simulink model "GMSK"  (R2024a)
settings: Solver=VariableStepAuto  StartTime=0.0  StopTime=4e-5  RelTol=1e-3
undefined symbols (not defined in the file or in its folder): DESIGN_CONST
libraries: dspfdesign x5, simulink x2, dspsigops x1, msbPllFoundation x1
settings Model: Creator=Sayantan  LastModifiedBy=Sayantan

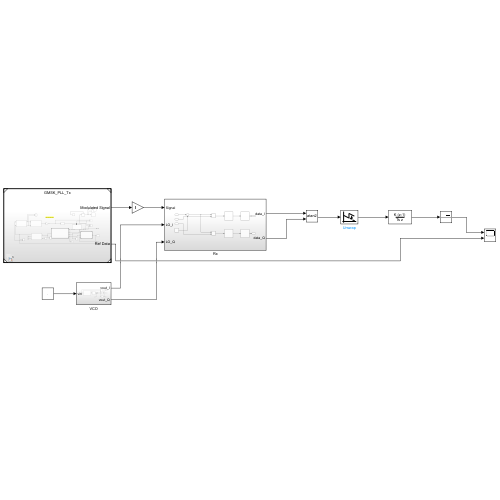
[thumbnail: Simulink's stored preview of the top-level diagram]
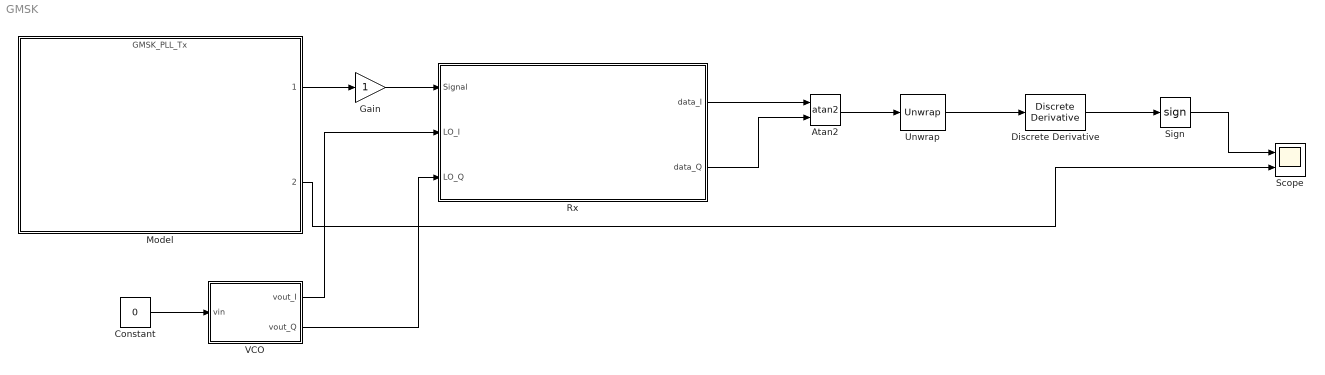
== system GMSK ==
  Atan2 : Trigonometry  Operator=atan2
  Constant : Constant  Value=0
  Discrete Derivative : simulink/Discrete/Discrete Derivative  gainval=1.0  ICPrevScaledInput=0.0  OutMin=[]  OutMax=[]  OutDataType=fixdt(1, 16)  OutScaling=2^-10  DoSatur=off
  Gain : Gain
  Model : ModelReference  ModelNameDialog=GMSK_PLL_Tx.slx  SimulationMode=Normal  ModelReferenceVersion=1.48
  Rx : Subsystem
  Scope : Scope  NumInputPorts=2
  Sign : Signum
  Unwrap : dspsigops/Unwrap  tol=pi  InputProcessing=Columns as channels (frame based)  running=off
  VCO : Subsystem
  wires:
  Gain/1 -> Rx/1(Signal)
  Model/1 -> Gain/1
  VCO/1(vout_I) -> Rx/2(LO_I)
  VCO/2(vout_Q) -> Rx/3(LO_Q)
  Model/2 -> Scope/2
  Rx/1(data_I) -> Atan2/1
  Rx/2(data_Q) -> Atan2/2
  Constant/1 -> VCO/1(vin)
  Atan2/1 -> Unwrap/1
  Sign/1 -> Scope/1
  Unwrap/1 -> Discrete Derivative/1
  Discrete Derivative/1 -> Sign/1

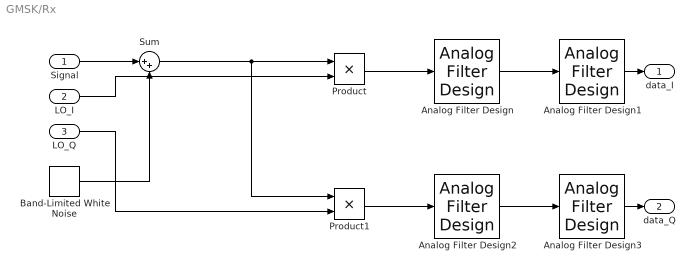
== system GMSK/Rx ==
  Signal : Inport
  LO_I : Inport  Port=2
  LO_Q : Inport  Port=3
  Analog Filter Design{,1..3} (4 alike) : dspfdesign/Analog Filter Design  method=Butterworth  filttype=Lowpass  N=1  Wlo=2*pi*(5e6)  Whi=80  Rp=2  Rs=40
  Band-Limited White Noise : simulink/Sources/Band-Limited White Noise  Cov=[0]  Ts=DESIGN_CONST.Tsim  seed=[23341]
  Product : Product
  Product1 : Product
  Sum : Sum  Inputs=|++
  data_I : Outport
  data_Q : Outport  Port=2
  wires:
  Analog Filter Design1/1 -> data_I/1
  Sum/1 -> Product1/1, Product/1
  Analog Filter Design/1 -> Analog Filter Design1/1
  Product/1 -> Analog Filter Design/1
  Analog Filter Design3/1 -> data_Q/1
  Band-Limited White Noise/1 -> Sum/2
  LO_I/1 -> Product/2
  Analog Filter Design2/1 -> Analog Filter Design3/1
  Product1/1 -> Analog Filter Design2/1
  Signal/1 -> Sum/1
  LO_Q/1 -> Product1/2

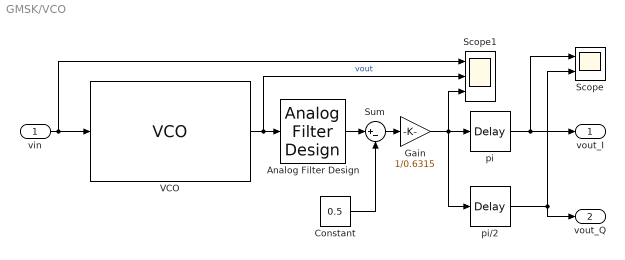
== system GMSK/VCO ==
  vin : Inport
  Analog Filter Design : dspfdesign/Analog Filter Design  method=Butterworth  filttype=Lowpass  N=8  Wlo=2*pi*1200e6  Whi=80  Rp=2  Rs=40
  Constant : Constant  Value=0.5
  Gain : Gain  Gain=1/0.6315
  Scope : Scope  NumInputPorts=2
  Scope1 : Scope  NumInputPorts=3
  Sum : Sum  Inputs=|+-
  VCO : msbPllFoundation/VCO  SpecifyUsing=Voltage sensitivity  Kvco=30e6  Fo=900e6  ControlVoltage=[-5 0 5]  OutputFrequency=[2e9 2.5e9 3e9]  Amplitude=1  ExtraBuffer=off  NBuffer=1000  AddPhaseNoise=on  Foffset=[1e6 (10^0.2)*1e6 sqrt(10)*1e6 10e6 100e6]  PhaseNoise=[-126.757 -126.775 -127.725 -140 -160]  MaxKvco=30000000
  pi : TransportDelay  DelayTime=2/(4*900e6)
  pi/2 : TransportDelay  DelayTime=1/(4*900e6)
  vout_I : Outport
  vout_Q : Outport  Port=2
  wires:
  vin/1 -> Scope1/1, VCO/1
  VCO/1 -> Scope1/2, Analog Filter Design/1  "vout"
  pi/1 -> Scope/1, vout_I/1
  pi/2/1 -> vout_Q/1, Scope/2
  Gain/1 -> Scope1/3, pi/2/1, pi/1
  Analog Filter Design/1 -> Sum/1
  Sum/1 -> Gain/1
  Constant/1 -> Sum/2
